simulink model "tau_4"  (R2019b)
settings: Solver=VariableStepAuto  StartTime=0.0  StopTime=25  RelTol=1e-3
model workspace (MAT data in the model file):
  k = 0.5
libraries: simulink x6
settings Model: Creator=Sergey  LastModifiedBy=Sergey

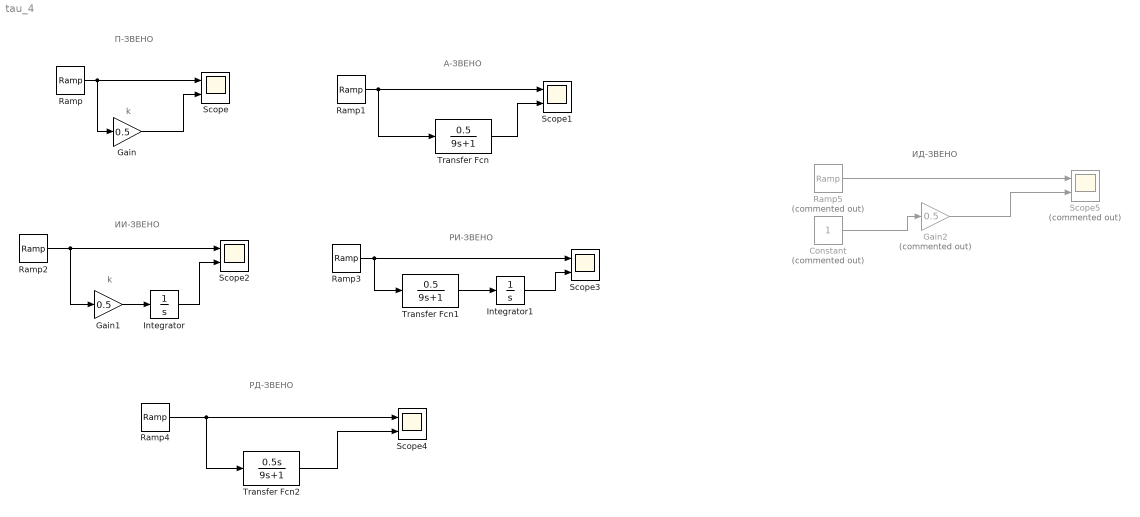
== system tau_4 ==
  note: ИД-ЗВЕНО
  note: РД-ЗВЕНО
  note: РИ-ЗВЕНО
  note: ИИ-ЗВЕНО
  note: А-ЗВЕНО
  note: П-ЗВЕНО
  note: k
  note: k
  Constant : Constant  Commented=on
  Gain : Gain  Gain=0.5
  Gain1 : Gain  Gain=0.5
  Gain2 : Gain  Commented=on  Gain=0.5
  Integrator : Integrator
  Integrator1 : Integrator
  Ramp{,1..4} (5 alike) : simulink/Sources/Ramp  slope=0  start=0  InitialOutput=1
  Ramp5 : simulink/Sources/Ramp  Commented=on  slope=0  start=0  InitialOutput=1
  Scope{,1..4} (5 alike) : Scope  NumInputPorts=2
  Scope5 : Scope  Commented=on  NumInputPorts=2
  Transfer Fcn : TransferFcn  Numerator=[0.5]  Denominator=[9 1]
  Transfer Fcn1 : TransferFcn  Numerator=[0.5]  Denominator=[9 1]
  Transfer Fcn2 : TransferFcn  Numerator=[0.5 0]  Denominator=[9 1]
  wires:
  Ramp/1 -> Gain/1, Scope/1
  Gain/1 -> Scope/2
  Ramp1/1 -> Transfer Fcn/1, Scope1/1
  Transfer Fcn/1 -> Scope1/2
  Gain1/1 -> Integrator/1
  Ramp2/1 -> Scope2/1, Gain1/1
  Integrator/1 -> Scope2/2
  Transfer Fcn1/1 -> Integrator1/1
  Ramp3/1 -> Transfer Fcn1/1, Scope3/1
  Integrator1/1 -> Scope3/2
  Ramp4/1 -> Transfer Fcn2/1, Scope4/1
  Transfer Fcn2/1 -> Scope4/2
  Gain2/1 -> Scope5/2
  Ramp5/1 -> Scope5/1
  Constant/1 -> Gain2/1
